simulink model "Q6"  (R2022a)
settings: Solver=VariableStepAuto  StartTime=0.0  StopTime=30  RelTol=1e-3
settings Model: Creator=chitn  LastModifiedBy=manan
settings DebuggingCC: UnconnectedInputMsg=warning  UnconnectedOutputMsg=warning  UnconnectedLineMsg=warning
settings RTWCC: DLArmComputeVersion=19.05

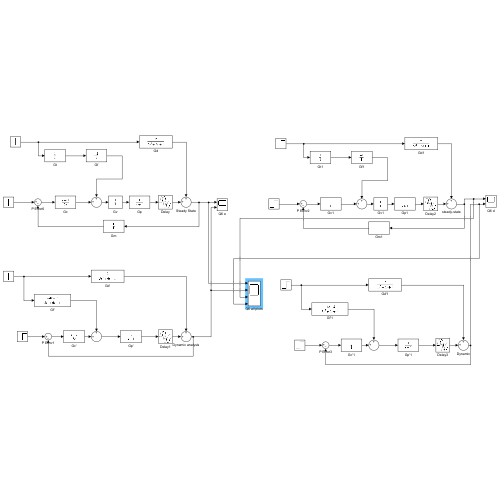
[thumbnail: Simulink's stored preview of the top-level diagram]
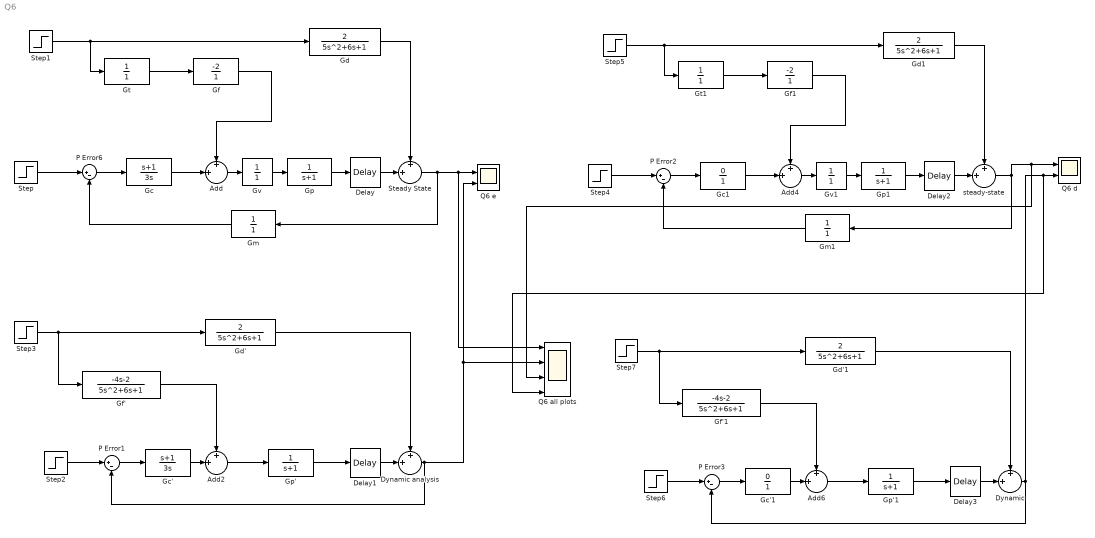
== system Q6 ==
  Add{,2,4,6} (4 alike) : Sum  Inputs=+|+||
  Delay{,1..3} (4 alike) : TransportDelay
  Dynamic : Sum  Inputs=+|+||
  Dynamic analysis : Sum  Inputs=+|+||
  Gc : TransferFcn  Numerator=[1 1]  Denominator=[3 0]
  Gc' : TransferFcn  Numerator=[1 1]  Denominator=[3 0]
  Gc'1 : TransferFcn  Numerator=0  Denominator=1
  Gc1 : TransferFcn  Numerator=0  Denominator=1
  Gd : TransferFcn  Numerator=2  Denominator=[5 6 1]
  Gd' : TransferFcn  Numerator=2  Denominator=[5 6 1]
  Gd'1 : TransferFcn  Numerator=2  Denominator=[5 6 1]
  Gd1 : TransferFcn  Numerator=2  Denominator=[5 6 1]
  Gf : TransferFcn  Numerator=[-2]  Denominator=[1]
  Gf' : TransferFcn  Numerator=[-4 -2]  Denominator=[5 6 1]
  Gf'1 : TransferFcn  Numerator=[-4 -2]  Denominator=[5 6 1]
  Gf1 : TransferFcn  Numerator=[-2]  Denominator=[1]
  Gm : TransferFcn  Numerator=1  Denominator=1
  Gm1 : TransferFcn  Numerator=1  Denominator=1
  Gp : TransferFcn  Denominator=[1 1]
  Gp' : TransferFcn  Denominator=[1 1]
  Gp'1 : TransferFcn  Denominator=[1 1]
  Gp1 : TransferFcn  Denominator=[1 1]
  Gt : TransferFcn  Numerator=1  Denominator=1
  Gt1 : TransferFcn  Numerator=1  Denominator=1
  Gv : TransferFcn  Numerator=1  Denominator=1
  Gv1 : TransferFcn  Numerator=1  Denominator=1
  P Error{1..3,6} (4 alike) : Sum  Inputs=|+-
  Q6 all plots : Scope  NumInputPorts=4
  Q6 d : Scope  NumInputPorts=2
  Q6 e : Scope  NumInputPorts=2
  Steady State : Sum  Inputs=+|+||
  Step{,1..7} (8 alike) : Step  SampleTime=0
  steady-state : Sum  Inputs=+|+||
  wires:
  Step1/1 -> Gd/1, Gt/1
  Step/1 -> P Error6/1
  P Error6/1 -> Gc/1
  Add/1 -> Gv/1
  Gp/1 -> Delay/1
  Gf/1 -> Add/1
  Steady State/1 -> Gm/1, Q6 all plots/1, Q6 e/1
  Delay/1 -> Steady State/2
  Step2/1 -> P Error1/1
  Delay1/1 -> Dynamic analysis/2
  Step3/1 -> Gf'/1, Gd'/1
  Gd'/1 -> Dynamic analysis/1
  Gp'/1 -> Delay1/1
  P Error1/1 -> Gc'/1
  Add2/1 -> Gp'/1
  Gf'/1 -> Add2/1
  Dynamic analysis/1 -> P Error1/2, Q6 e/2, Q6 all plots/2
  Gc'/1 -> Add2/2
  Gc/1 -> Add/2
  Gd/1 -> Steady State/1
  Gt/1 -> Gf/1
  Gm/1 -> P Error6/2
  Gv/1 -> Gp/1
  Gv1/1 -> Gp1/1
  Gt1/1 -> Gf1/1
  Gc1/1 -> Add4/2
  Step4/1 -> P Error2/1
  Delay2/1 -> steady-state/2
  P Error2/1 -> Gc1/1
  Add4/1 -> Gv1/1
  steady-state/1 -> Q6 all plots/3, Q6 d/1, Gm1/1
  Gf1/1 -> Add4/1
  Gp1/1 -> Delay2/1
  Step5/1 -> Gd1/1, Gt1/1
  Gd1/1 -> steady-state/1
  Gm1/1 -> P Error2/2
  Gc'1/1 -> Add6/2
  Dynamic/1 -> Q6 all plots/4, Q6 d/2, P Error3/2
  Step7/1 -> Gf'1/1, Gd'1/1
  Gp'1/1 -> Delay3/1
  Gf'1/1 -> Add6/1
  Add6/1 -> Gp'1/1
  Step6/1 -> P Error3/1
  P Error3/1 -> Gc'1/1
  Gd'1/1 -> Dynamic/1
  Delay3/1 -> Dynamic/2
